simulink model "part_5"  (R2017a)
settings: Solver=VariableStepAuto  StartTime=0.0  StopTime=10.0  RelTol=1e-3
settings Model: Creator=malifarah  LastModifiedBy=malifarah

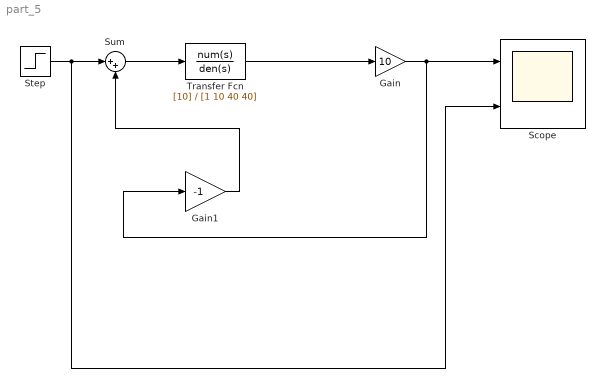
== system part_5 ==
  Gain : Gain  Gain=10
  Gain1 : Gain  Gain=-1
  Scope : Scope  NumInputPorts=2
  Step : Step  SampleTime=0
  Sum : Sum  Inputs=|++
  Transfer Fcn : TransferFcn  Numerator=[10]  Denominator=[1 10 40 40]
  wires:
  Step/1 -> Scope/2, Sum/1
  Transfer Fcn/1 -> Gain/1
  Sum/1 -> Transfer Fcn/1
  Gain1/1 -> Sum/2
  Gain/1 -> Gain1/1, Scope/1
